simulink model "pow_u_v"  (Simulink 6.2)
settings: Solver=FixedStepDiscrete  StartTime=0.0  StopTime=10.0  RelTol=1e-3
settings Model: LastModifiedBy=Bo
settings DebuggingCC: SolverPrmCheckMsg=warning

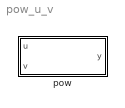
== system pow_u_v ==
  pow : Subsystem  Description=u^v

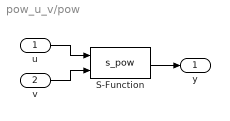
== system pow_u_v/pow ==
  u : Inport  Port=1  LatchInput=off
  v : Inport  Port=2  PortDimensions=1  LatchInput=off
  S-Function : S-Function  FunctionName=s_pow
  y : Outport
  wires:
  u/1 -> S-Function/1
  v/1 -> S-Function/2
  S-Function/1 -> y/1
